simulink model "power_window_controller"  (R2014b)
settings: Solver=FixedStepDiscrete  StartTime=0.0  StopTime=10.0  FixedStep=0.1  RelTol=1e-3
settings Model: Creator=z2akhtar  LastModifiedBy=z2akhtar
settings OptimizationCC: InlineParams=on  ExpressionDepthLimit=2147483647  ZeroExternalMemoryAtStartup=off  ZeroInternalMemoryAtStartup=off  OptimizeModelRefInitCode=on  LifeSpan=1
settings DebuggingCC: ModelReferenceSymbolNameMessage=none  StateNameClashWarn=warning
settings ModelReferenceCC: UpdateModelReferenceTargets=IfOutOfDate
settings RTWCC: SystemTargetFile=autosar.tlc  GenCodeOnly=on  TemplateMakefile=ert_default_tmf  Description=AUTOSAR  ProcessScript=autosar_make_rtw_hook
settings CodeAppCC: IgnoreCustomStorageClasses=off
settings STFCustomTargetCC: ParMdlRefBuildCompliant=on  CompOptLevelCompliant=on  IncludeMdlTerminateFcn=off  CombineOutputUpdateFcns=on  SuppressErrorStatus=on  ERTFirstTimeCompliant=on  ERTCustomFileBanners=on  SupportNonFinite=off  SupportComplex=off  SupportContinuousTime=off  SupportNonInlinedSFcns=off  MATLABClassNameForMDSCustomization=Simulink.SoftwareTarget.ERTCustomization  AutosarCompliant=on  GRTInterface=off  SystemTargetFile=autosar.tlc
settings ERTTargetCC: ConcurrentExecutionCompliant=off  IncludeMdlTerminateFcn=off  SuppressErrorStatus=on  SupportNonFinite=off  SupportComplex=off  ModelStepFunctionPrototypeControlCompliant=off  CPPClassGenCompliant=off  AutosarCompliant=on  InlinedParameterPlacement=NonHierarchical  ERTCustomFileTemplate=example_file_process.tlc

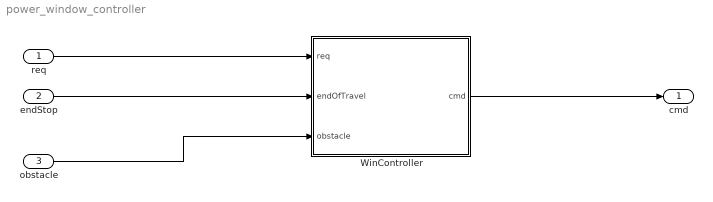
== system power_window_controller ==
  req : Inport  OutDataTypeStr=uint8
  endStop : Inport  Port=2  OutDataTypeStr=boolean
  obstacle : Inport  Port=3  OutDataTypeStr=boolean
  WinController : Stateflow chart
  cmd : Outport  OutDataTypeStr=uint8
  wires:
  endStop/1 -> WinController/2(endOfTravel)
  obstacle/1 -> WinController/3(obstacle)
  WinController/1(cmd) -> cmd/1
  req/1 -> WinController/1(req)

== stateflow chart power_window_controller/WinController ==
  state winStates
    state Stopped
      en: cmd = 0;
      state unknownPos
      state fullyClosed
      state fullyOpen
      state partiallyOpen
      (default) -> unknownPos
      unknownPos -> partiallyOpen
      partiallyOpen -> (junction 104)
    state movingUp
      en: cmd = 2;
      state movingUpBsc
      state movingUpX
        state mux_pp
        state mux_ppo
        (default) -> mux_ppo
        mux_ppo -> mux_pp : [req ~= 4]
      (default) -> movingUpBsc
      movingUpBsc -> movingUpX [order 1] : [req == 4]
    state movingDown
      en: cmd = 1;
      state movingDownBsc
      state movingDownX
      (default) -> movingDownBsc
      movingDownBsc -> movingDownX [order 1] : [req == 3]
    state retracting
      en: cmd = 1;
    state coolDown
      en: cmd = 0;
    (default) -> Stopped
    coolDown -> Stopped : [req == 0]
    movingUp -> fullyClosed [order 1] : [endOfTravel  == 1]
    fullyClosed -> (junction 123) [order 1] : [req == 1]
    fullyClosed -> (junction 72) [order 2] : [req==3]
    (junction 117) -> fullyOpen
    fullyOpen -> (junction 128) [order 2] : [req == 2]
    fullyOpen -> (junction 46) [order 1] : [req == 4]
    movingUpBsc -> partiallyOpen [order 2] : [(req == 0)]
    movingDownBsc -> partiallyOpen [order 2] : [req == 0]
    (junction 104) -> (junction 123) [order 2] : [req == 1]
    (junction 104) -> (junction 128) [order 1] : [req == 2]
    (junction 104) -> (junction 46) [order 4] : [req == 4]
    (junction 104) -> (junction 72) [order 3] : [req == 3]
    (junction 123) -> movingDown
    (junction 128) -> movingUp
    movingDown -> (junction 117) [order 1] : [endOfTravel]
    retracting -> (junction 117) : [endOfTravel]
    (junction 71) -> movingDownBsc
    movingUp -> (junction 71) [order 3] : [req == 1]
    movingDown -> (junction 73) [order 4] : [req == 2]
    (junction 73) -> movingUpBsc
    (junction 72) -> movingDownX
    movingUp -> (junction 72) [order 4] : [req == 3]
    movingDown -> (junction 46) [order 2] : [req == 4]
    (junction 46) -> movingUpX
    mux_pp -> (junction 39) : [obstacle == 1]
    movingDown -> coolDown [order 3] : [after(10, sec)]
    movingUp -> coolDown [order 2] : [after(10, sec)]
    (junction 39) -> retracting
  data: req input uint8; endOfTravel input boolean; obstacle input boolean; cmd output uint8
